simulink model "MOTOR_POSITION_CONTROL"  (R2020b)
settings: Solver=ode15s  StartTime=0.0  StopTime=0.08  RelTol=1e-3
PreLoadFcn:
  | J=3.2284E-6;
  | b=3.5077E-6;
  | K=0.0274;
  | R=4;
  | L=2.75E-6;
settings Model: DataDictionary=DataDict_Motor_position.sldd  Creator=intel  LastModifiedBy=intel
settings DebuggingCC: AlgebraicLoopMsg=none

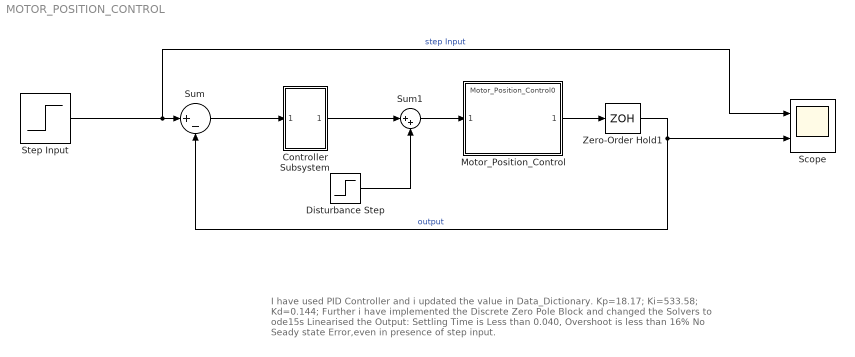
== system MOTOR_POSITION_CONTROL ==
  note: I have used PID Controller and i updated the value in Data_Dictionary.
      | Kp=18.17;
      | Ki=533.58;
      | Kd=0.144;
      |
      | Further i have implemented the Discrete Zero Pole Block and changed the Solvers to ode15s
      | Linearised the Output:
      | Settling Time is Less than 0.040,
      | Overshoot is less than 16%
      | No Seady state Error,even in presence of step input.
  " Step Input" : Step  Time=0  SampleTime=0
  " Zero-Order Hold1" : ZeroOrderHold  SampleTime=0.001
  Controller Subsystem : Subsystem
  Disturbance Step : Step  Time=0.03  SampleTime=0
  Motor_Position_Control : ModelReference  ModelNameDialog=Motor_Position_Control0  ModelReferenceVersion=1.7
  Scope : Scope  NumInputPorts=2
  Sum : Sum  Inputs=|+-
  Sum1 : Sum  Inputs=|++
  wires:
  " Step Input"/1 -> Scope/1, Sum/1  "step Input"
  " Zero-Order Hold1"/1 -> Scope/2, Sum/2  "output"
  Motor_Position_Control/1 -> " Zero-Order Hold1"/1
  Sum1/1 -> Motor_Position_Control/1
  Disturbance Step/1 -> Sum1/2
  Sum/1 -> Controller Subsystem/1(In1)
  Controller Subsystem/1(Out1) -> Sum1/1

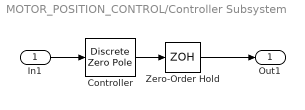
== system MOTOR_POSITION_CONTROL/Controller Subsystem ==
  In1 : Inport
  " Zero-Order Hold" : ZeroOrderHold  SampleTime=0.001
  Controller : DiscreteZeroPole  Zeros=[0.95 0.80 0.80]  Poles=[-0.98 0.6 1]  Gain=800  SampleTime=0.001
  Out1 : Outport
  wires:
  " Zero-Order Hold"/1 -> Out1/1
  Controller/1 -> " Zero-Order Hold"/1
  In1/1 -> Controller/1
